simulink model "IP_LinearSys_Openloop_KF"  (R2015a)
settings: Solver=ode5  StartTime=0.0  StopTime=10.0  FixedStep=0.01  RelTol=1e-3
undefined symbols (not defined in the file): A, B, C, Continuous, D, sigbuilder_block, Time, Ts
libraries: simulink x2, ctrlSharedLib x1
settings Model: Creator=Fares  LastModifiedBy=Fares

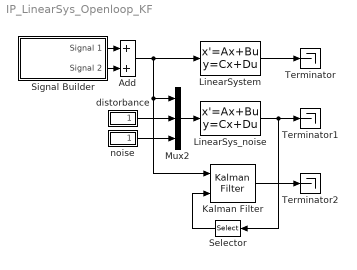
== system IP_LinearSys_Openloop_KF ==
  Add : Sum
  Kalman Filter : ctrlSharedLib/Kalman Filter  TimeDomain=Continuous-Time  UseCurrentEstimator=on  ModelSource=Individual A, B, C, D matrices  ModelSourceVariable=ss(A,B,C,D,Ts)  A=A  B=B  C=C  D=D  NumberOfStates=1  NumberOfInputs=1  NumberOfOutputs=1  InitialEstimateSource=Dialog  X0=[0; 0; 0; 0]  P0=10  UseK=off  UseGH=off  NumberOfProcessNoiseInputs=1  G=1  TimeInvariantG=on  H=0  TimeInvariantH=on  Q=diag([1e-03 1e-03 0.1 0.1])  TimeInvariantQ=on  R=1e-04  TimeInvariantR=on  N=0  TimeInvariantN=on  AddInputPort=on  AddEnablePort=off  ExternalReset=none  OutputEstimatedY=off  OutputP=off  Ts=-1
  LinearSys_noise : StateSpace  A=A  B=BF  C=C  D=DF  X0=[0; 0; 0; 0]  mask(SS MASK){}
      mask init:
      | mc = 1.12;
      | mpw = 0.095;
      | mps = 0.025;
      | l = 0.033245968;
      | fc = 2.53165; % FS = 2.53165; FC = 2.28133
      | fp = 0.000107443;
      | J = 0.013935418;
      | g = 9.81;
      | vf = 9.4/2.5; %Voltage to Motor Force ratio
      | mp = mpw + mps;
      | a = l^2 + J/(mc + mp);
      | mu = (mc + mp)*l;
      | 
      | % theta 0 in upward position
      | % theta pi in downward position
      | s = -1; % 1 when upward  -1 when downward
      | 
      | A = [0          0              1               0;
      |      0          0              0               1;
      |      0      (l*mu*g)/J    -(a*fc)/J    -(l*fp)/J;
      |      0      s*(mu*g)/J    -s*(l*fc)/J    -(fp)/J];
      |  
      | B = [         0;
      |               0;
      |        (vf*a)/J;
      |       (s*vf*l)/J];
      |   
      | C = [1 0 0 0;
      |      0 1 0 0;
      |      0 0 1 0;
      |      0 0 0 1];
      |  
      | D = [0;
      |      0;
      |      0;
      |      0];
      |  
      | G = eye(4);
      | H = [1;
      |      0;
      |      0;
      |      0];
      |  
      | BF = [B G zeros(4,1)];
      | DF = [D zeros(4,4) H];
  LinearSystem : StateSpace  A=A  B=B  C=C  D=D  X0=[0; 0; 0; 0]  mask(SS MASK){}
      mask init:
      | mc = 1.12;
      | mpw = 0.095;
      | mps = 0.025;
      | l = 0.033245968;
      | fc = 2.53165; % FS = 2.53165; FC = 2.28133
      | fp = 0.000107443;
      | J = 0.013935418;
      | g = 9.81;
      | vf = 9.4/2.5; %Voltage to Motor Force ratio
      | mp = mpw + mps;
      | a = l^2 + J/(mc + mp);
      | mu = (mc + mp)*l;
      | 
      | % theta 0 in upward position
      | % theta pi in downward position
      | s = -1; % 1 when upward  -1 when downward
      | 
      | A = [0          0              1               0;
      |      0          0              0               1;
      |      0      (l*mu*g)/J    -(a*fc)/J    -(l*fp)/J;
      |      0      s*(mu*g)/J    -s*(l*fc)/J    -(fp)/J];
      |  
      | B = [         0;
      |               0;
      |        (vf*a)/J;
      |       (s*vf*l)/J];
      |   
      | C = [1 0 0 0;
      |      0 1 0 0;
      |      0 0 1 0;
      |      0 0 0 1];
      |  
      | D = [0;
      |      0;
      |      0;
      |      0];
  Mux2 : Mux  Inputs=3
  Selector : Selector  InputPortWidth=4  Indices=[1]
  Signal Builder : Subsystem  Tag=STV Subsys  LoadFcn=sigbuilder_block('load');  StartFcn=sigbuilder_block('start');  StopFcn=sigbuilder_block('stop');  ClipboardFcn=sigbuilder_block('clipboard');  mask(Sigbuilder block){}
      mask help: Simulink:masks:SigbuilderBlock_MD
      mask init:
      | if ~strcmp(get_param(bdroot(gcbh),'SimulationStatus'),'stopped') tuvar = sigbuilder_block('maskInit'); end
      settings: CopyFcn=sigbuilder_block('copy');  DeleteFcn=sigbuilder_block('delete');  ModelCloseFcn=sigbuilder_block('modelClose');  PreSaveFcn=sigbuilder_block('preSave');  PauseFcn=sigbuilder_block('pause');  ContinueFcn=sigbuilder_block('continue');  NameChangeFcn=sigbuilder_block('namechange');  OpenFcn=sigbuilder_block('open',[437.6 199.2 550.4 400 ]);  CloseFcn=sigbuilder_block('close');
      mask Display: plot(0, 0, 100, 100,[2, 2, 32, 32, 2], [68, 8, 8, 68, 68],[32, 2], [38, 38], [32, 19, 2],[53, 60, 44], [32, 17, 17, 2],[16, 16, 31, 31]);txt = getActiveGroup(gcbh);text(2, 100, txt,'verticalAlignment', 'top');
  Terminator : Terminator
  Terminator1 : Terminator
  Terminator2 : Terminator
  distorbance : Subsystem
  noise : Subsystem
  wires:
  Signal Builder/1(Signal 1) -> Add/1
  LinearSystem/1 -> Terminator/1
  Signal Builder/2(Signal 2) -> Add/2
  distorbance/1(Out1) -> Mux2/2
  noise/1(Out1) -> Mux2/3
  Mux2/1 -> LinearSys_noise/1
  LinearSys_noise/1 -> Selector/1, Terminator1/1
  Kalman Filter/1 -> Terminator2/1
  Add/1 -> LinearSystem/1, Kalman Filter/1, Mux2/1
  Selector/1 -> Kalman Filter/2

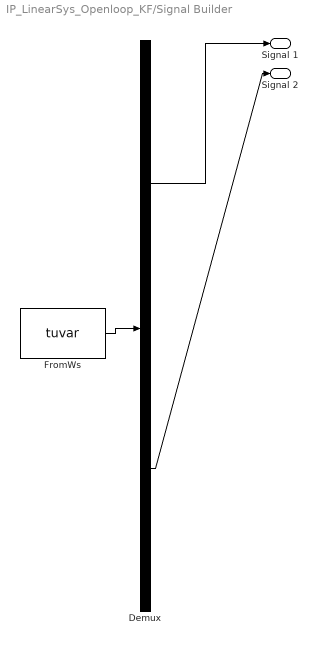
== system IP_LinearSys_Openloop_KF/Signal Builder ==
  Demux : Demux  Tag=STV Demux  Outputs=2
  FromWs : FromWorkspace  Tag=STV FromWs  VariableName=tuvar  SampleTime=0
      SigBuilderData=|
      | common.afterFinalStr = 'Extrapolate'
      | common.sampleTime = 0
      | dataSet.timeRange = [0 10]
      | dataSet.name = 'Group 1'
      | sbobj.Groups.Name = 'Group 1'
      | sbobj.Groups.Signals(1).Name = 'Signal 1'
      | sbobj.Groups.Signals(1).XData = [0 1 1 1.1 1.1 10]
      | sbobj.Groups.Signals(1).YData = [0 0 2 2 0 0]
      | sbobj.Groups.Signals(2).Name = 'Signal 2'
      | sbobj.Groups.Signals(2).XData = [0 5 5 5.1 5.1 10]
      | sbobj.Groups.Signals(2).YData = [0 0 -2 -2 0 0]
  Signal 1 : Outport  Tag=STV Outport
  Signal 2 : Outport  Tag=STV Outport  Port=2
  wires:
  Demux/2 -> Signal 2/1
  FromWs/1 -> Demux/1
  Demux/1 -> Signal 1/1

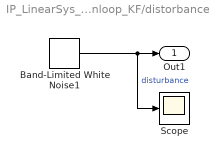
== system IP_LinearSys_Openloop_KF/distorbance ==
  Band-Limited White Noise1 : simulink/Sources/Band-Limited White Noise  Cov=[0 0 0.1*0.01 0.1*0.01]  Ts=0.01  seed=[23341]
  Scope : Scope
      settings: SaveName=noise
  Out1 : Outport
  wires:
  Band-Limited White Noise1/1 -> Scope/1, Out1/1  "disturbance"

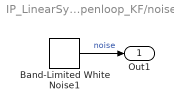
== system IP_LinearSys_Openloop_KF/noise ==
  Band-Limited White Noise1 : simulink/Sources/Band-Limited White Noise  Cov=[1e-4*0.01]  Ts=0.01  seed=[23341]
  Out1 : Outport
  wires:
  Band-Limited White Noise1/1 -> Out1/1  "noise"
